simulink model "Hill_type_muscleModel_RampTest"  (R2019b)
settings: Solver=VariableStepAuto  StartTime=0.0  StopTime=20  RelTol=1e-3
values from neighbouring files (symbols this model uses):
  a0 = 0.165    [HillTypeMuscleModel_params_debug.m]
  activation_freq = freq(n)    [HillTypeMuscleModel_params_debug.m]
  beta = 0.703    [HillTypeMuscleModel_params_debug.m]
  F0 = 150/1000    (= 0.15)    [HillTypeMuscleModel_params_debug.m]
  g_scale = 2.0    (= 2)    [HillTypeMuscleModel_params_debug.m]
  K_t = 5*F0/L_0    (= 47.7664412091)    [HillTypeMuscleModel_params_debug.m]
  L_m_0 = L_mto    (= 0.0183)    [HillTypeMuscleModel_params_debug.m]
  L_mto = 18.3/1000    (= 0.0183)    [HillTypeMuscleModel_params_debug.m]
  L_st = 0    [HillTypeMuscleModel_params_debug.m]
  tau = 2.45    [HillTypeMuscleModel_params_debug.m]
  v_max = 0.007    [HillTypeMuscleModel_params_debug.m]
undefined symbols (not defined in the file or in its folder): Ramp
libraries: simulink x1
settings Model: Creator=mecha  LastModifiedBy=mecha

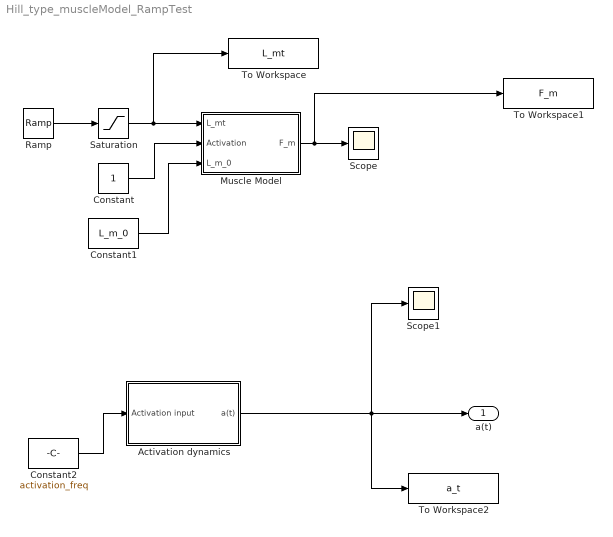
== system Hill_type_muscleModel_RampTest ==
  Activation dynamics : Subsystem
  Constant : Constant
  Constant1 : Constant  Value=L_m_0
  Constant2 : Constant  Value=activation_freq
  Muscle Model : Subsystem
  Ramp : simulink/Sources/Ramp  slope=Ramp.rate  start=Ramp.start_time  InitialOutput=Ramp.initial_output
  Saturation : Saturate  UpperLimit=Ramp.L_max  LowerLimit=Ramp.L_min
  Scope : Scope
  Scope1 : Scope
  To Workspace : ToWorkspace  VariableName=L_mt  SaveFormat=Timeseries  SampleTime=-1
  To Workspace1 : ToWorkspace  VariableName=F_m  SaveFormat=Timeseries  SampleTime=-1
  To Workspace2 : ToWorkspace  VariableName=a_t  SaveFormat=Timeseries  SampleTime=-1
  "a(t) " : Outport
  wires:
  Muscle Model/1(F_m) -> To Workspace1/1, Scope/1
  Saturation/1 -> To Workspace/1, Muscle Model/1(L_mt)
  Ramp/1 -> Saturation/1
  Constant1/1 -> Muscle Model/3(L_m_0)
  Constant2/1 -> Activation dynamics/1(Activation input)
  Activation dynamics/1("a(t) ") -> To Workspace2/1, Scope1/1, "a(t) "/1
  Constant/1 -> Muscle Model/2(Activation)

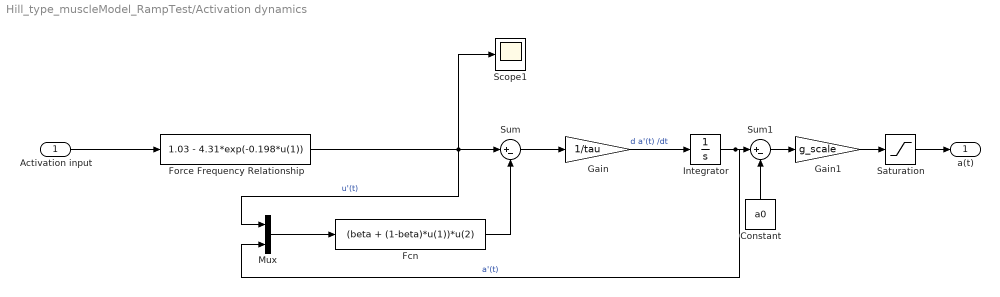
== system Hill_type_muscleModel_RampTest/Activation dynamics ==
  Activation input : Inport
  Constant : Constant  Value=a0
  Fcn : Fcn  Expr=(beta + (1-beta)*u(1))*u(2)
  Force Frequency Relationship : Fcn  Expr=1.03 - 4.31*exp(-0.198*u(1))
  Gain : Gain  Gain=1/tau
  Gain1 : Gain  Gain=g_scale
  Integrator : Integrator
  Mux : Mux  Inputs=2
  Saturation : Saturate  UpperLimit=2  LowerLimit=0
  Scope1 : Scope
  Sum : Sum  Inputs=|+-
  Sum1 : Sum  Inputs=|+-
  "a(t) " : Outport
  wires:
  Activation input/1 -> Force Frequency Relationship/1
  Sum/1 -> Gain/1
  Force Frequency Relationship/1 -> Scope1/1, Mux/1, Sum/1  "u'(t)"
  Integrator/1 -> Mux/2, Sum1/1  "a'(t)"
  Mux/1 -> Fcn/1
  Gain/1 -> Integrator/1  "d a'(t) /dt"
  Fcn/1 -> Sum/2
  Gain1/1 -> Saturation/1
  Sum1/1 -> Gain1/1
  Constant/1 -> Sum1/2
  Saturation/1 -> "a(t) "/1

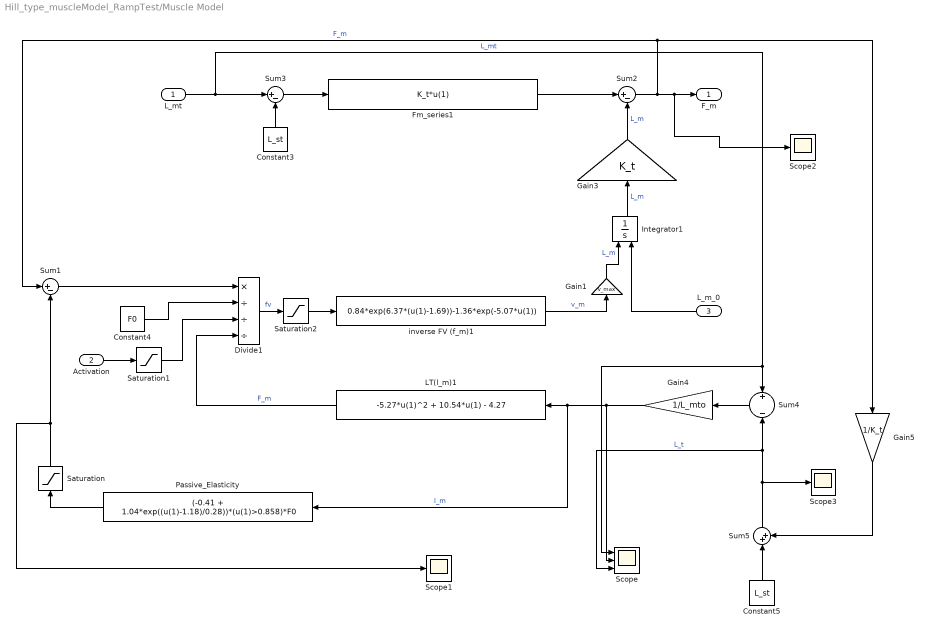
== system Hill_type_muscleModel_RampTest/Muscle Model ==
  L_mt : Inport
  Activation : Inport  Port=2
  L_m_0 : Inport  Port=3
  Constant3 : Constant  Value=L_st
  Constant4 : Constant  Value=F0
  Constant5 : Constant  Value=L_st
  Divide1 : Product  Inputs=*///
  Fm_series1 : Fcn  Expr=K_t*u(1)
  Gain1 : Gain  Gain=v_max
  Gain3 : Gain  Gain=K_t
  Gain4 : Gain  Gain=1/L_mto
  Gain5 : Gain  Gain=1/K_t
  Integrator1 : Integrator  InitialConditionSource=external
  LT(l_m)1 : Fcn  Expr=-5.27*u(1)^2 + 10.54*u(1) - 4.27
  Passive_Elasticity : Fcn  Expr=(-0.41 + 1.04*exp((u(1)-1.18)/0.28))*(u(1)>0.858)*F0
  Saturation : Saturate  UpperLimit=inf  LowerLimit=0
  Saturation1 : Saturate  UpperLimit=1  LowerLimit=0.0001
  Saturation2 : Saturate  UpperLimit=2  LowerLimit=0
  Scope : Scope  NumInputPorts=3
  Scope1 : Scope
  Scope2 : Scope
  Scope3 : Scope
  Sum1 : Sum  Inputs=|+-
  Sum2 : Sum  Inputs=|+-
  Sum3 : Sum  Inputs=|+-
  Sum4 : Sum  Inputs=+||-
  Sum5 : Sum  Inputs=|++
  inverse FV (f_m)1 : Fcn  Expr=0.84*exp(6.37*(u(1)-1.69))-1.36*exp(-5.07*u(1))
  F_m : Outport
  wires:
  Fm_series1/1 -> Sum2/1
  Gain3/1 -> Sum2/2  "L_m"
  Sum3/1 -> Fm_series1/1
  Constant3/1 -> Sum3/2
  Divide1/1 -> Saturation2/1  "fv"
  Sum2/1 -> Sum1/1, Gain5/1, Scope2/1, F_m/1  "F_m"
  Constant4/1 -> Divide1/2
  Activation/1 -> Saturation1/1
  LT(l_m)1/1 -> Divide1/4  "F_m"
  L_mt/1 -> Scope/1, Sum4/1, Sum3/1  "L_mt"
  Gain4/1 -> Scope/2, Passive_Elasticity/1, LT(l_m)1/1  "l_m"
  Sum4/1 -> Gain4/1
  Sum5/1 -> Scope3/1, Sum4/2, Scope/3  "L_t"
  Gain5/1 -> Sum5/2
  Constant5/1 -> Sum5/1
  L_m_0/1 -> Integrator1/2
  Integrator1/1 -> Gain3/1  "L_m"
  Gain1/1 -> Integrator1/1  "L_m"
  inverse FV (f_m)1/1 -> Gain1/1  "v_m"
  Sum1/1 -> Divide1/1
  Passive_Elasticity/1 -> Saturation/1
  Saturation1/1 -> Divide1/3
  Saturation2/1 -> inverse FV (f_m)1/1
  Saturation/1 -> Scope1/1, Sum1/2
